simulink library "Lib_Analytic"  (R2019b)
settings: Solver=VariableStepAuto  StartTime=0.0  StopTime=10.0  RelTol=1e-3
undefined symbols (not defined in the file): SJac_Per_M, SNR_DX_M, SNR_IC_M, SNR_Mn_M, SNR_Mx_M
libraries: simulink x2
(part 2 of 2)

== system Lib_Analytic/Solvers/SS NR Solver w JacobianCalc/JacCalc w Reset ==
  f(x) : Inport  PortDimensions=length(SNR_IC_M)
  CCnd : Inport  Port=2  PortDimensions=1
  x(n+1) : Inport  Port=3  PortDimensions=length(SNR_IC_M)
  Enable : EnablePort
  Abs : Abs
  Constant : Constant  Value=SNR_IC_M
  JC_Reset counter : Subsystem
  Jacobian Calculator : Subsystem  TreatAsAtomicUnit=on  mask(T-MATS: Jacobian Calculator Library Block){N_Per_M=SJac_Per_M}
      mask prompts: N_Per_M "N_Per_M - Perturbations (nxm)"
      mask help:
      | The Jacobian Calculator block calculates the Jabobian of the system by perturbing the system around an initial point and calculating the gradient for each perturbation. This module will run once on start up and then again only if the reset is pressed.
      | Below: n (rows) is the number of times each independent will be perturbed and m (columns) is the number of inputs.
      mask Help: web(which('NumMthd_TMATS_JC.html'),'-helpbrowser')
  Product : Product  RndMeth=Zero
  Switch : Switch  Criteria=u2 ~= 0  Threshold=1
  Terminator3 : Terminator
  Unit Delay2 : UnitDelay  InitialCondition=SNR_IC_M./abs(SNR_IC_M)  SampleTime=-1  HasFrameUpgradeWarning=on
  X_out : Outport  PortDimensions=length(SNR_IC_M)
  JC_Active : Outport  Port=2  PortDimensions=1
  inv(J) : Outport  Port=3  PortDimensions=[length(SNR_IC_M),length(SNR_IC_M)]
  J : Outport  Port=4  PortDimensions=[length(SNR_IC_M),length(SNR_IC_M)]
  JacFailed : Outport  Port=5  PortDimensions=1
  wires:
  Jacobian Calculator/3(Iteration) -> Terminator3/1
  Jacobian Calculator/2(x_p) -> Switch/1
  Jacobian Calculator/4(Active) -> [JC_Active], JC_Active/1
  Unit Delay2/1 -> Switch/3, Jacobian Calculator/3(Xo)
  Constant/1 -> Abs/1
  Jacobian Calculator/5(inv(J)) -> inv(J)/1
  [JC_Active] -> JC_Reset counter/1(Reset Counter)
  Switch/1 -> Product/1
  Jacobian Calculator/1(J) -> J/1  "J"
  Product/1 -> X_out/1
  JC_Reset counter/1(JC_Reset) -> Jacobian Calculator/1(Reset)
  x(n+1)/1 -> Unit Delay2/1
  CCnd/1 -> JC_Reset counter/2(Count Condition)
  [JC_Active] -> Switch/2
  f(x)/1 -> Jacobian Calculator/2(f(x_p))
  Jacobian Calculator/6(JacFailed) -> JacFailed/1
  Abs/1 -> Product/2

== system Lib_Analytic/Solvers/SS NR Solver w JacobianCalc/NewRaph w Cond ==
  f(x(n)) : Inport  PortDimensions=length(SNR_IC_M)
  JC_Active : Inport  Port=2  PortDimensions=1
  inv(f'x(n)) : Inport  Port=3  PortDimensions=[length(SNR_IC_M),length(SNR_IC_M)]
  Enable : EnablePort
  Logical Operator : Logic  Operator=NOT  AllPortsSameDT=off  OutDataTypeStr=boolean
  Logical Operator1 : Logic  AllPortsSameDT=off  OutDataTypeStr=boolean
  Logical Operator2 : Logic  Operator=NOT  AllPortsSameDT=off  OutDataTypeStr=boolean
  Newton Raphson Solver : Subsystem  TreatAsAtomicUnit=on  mask(T-MATS: Newton Raphson Solver Library Block){NR_IC_M=SNR_IC_M./abs(SNR_IC_M), NR_dx_Lim_M=SNR_DX_M, NR_Mx_Lim_M=SNR_Mx_M./abs(SNR_IC_M), NR_Mn_Lim_M=SNR_Mn_M./abs(SNR_IC_M), BlkNm_M=double(gcb)}
      mask prompts: NR_IC_M "NR_IC_M - Initial Conditions of Newton Raphson (mx1)"; NR_dx_Lim_M "NR_dx_Lim_M - Newton Raphson step size limit (%) (1x1)"; NR_Mx_Lim_M "NR_Mx_Lim_M - Max limit (1x1 or mx1)"; NR_Mn_Lim_M "NR_Mn_Lim_M - Min Limit (1x1 or mx1)"; BlkNm_M "BlkNm_M - Block Name"
      mask help:
      | Newton Raphson Solver:
      |
      | x(n+1) = x(n) - inverse(f'(x(n)))*f(x(n))
      |
      | Note:
      | inverse(f'(x(n))) is an m x m matrix and f(x(n)) is an m x 1 matrix
      | where m is the length of the initial conditions matrix and number of system independents.
      mask init: same as Lib_Analytic/Numerical Methods/Newton Raphson Solver
      mask Help: web(which('NumMthd_TMATS_NRS.html'),'-helpbrowser')
  Terminator : Terminator
  conditions : Subsystem
  Converged : Outport  PortDimensions={1,[length(SNR_IC_M),length(SNR_IC_M)]}
  CCnd : Outport  Port=2  PortDimensions=1
  x(n+1) : Outport  Port=3  PortDimensions=length(SNR_IC_M)
  wires:
  Logical Operator/1 -> Logical Operator1/1
  Logical Operator1/1 -> Newton Raphson Solver/1(Enable)
  conditions/1(Condition) -> Logical Operator2/1, CCnd/1, Logical Operator1/2
  Logical Operator2/1 -> Converged/1  "Converged"
  JC_Active/1 -> Logical Operator/1
  inv(f'x(n))/1 -> Newton Raphson Solver/2(inv(f'(x(n))))
  Newton Raphson Solver/1(x(n)) -> Terminator/1
  Newton Raphson Solver/2(x(n+1)) -> x(n+1)/1
  f(x(n))/1 -> conditions/1(f(x)), Newton Raphson Solver/3(f(x(n)))

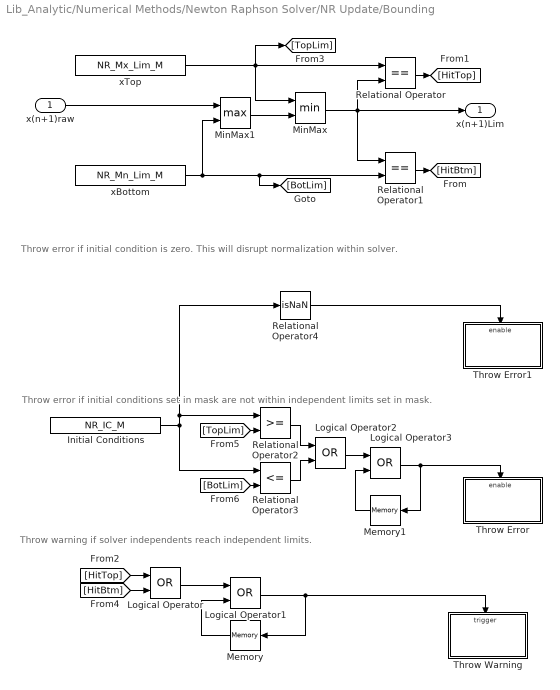
== system Lib_Analytic/Numerical Methods/Newton Raphson Solver/NR Update/Bounding ==
  note: Throw warning if solver independents reach independent limits.
  note: Throw error if initial conditions set in mask are not within independent limits set in mask.
  note: Throw error if initial condition is zero. This will disrupt normalization within solver.
  x(n+1)raw : Inport
  Initial Conditions : Constant  Value=NR_IC_M
  Logical Operator{,1..3} (4 alike) : Logic  Operator=OR  AllPortsSameDT=off  OutDataTypeStr=boolean
  Memory : Memory  InheritSampleTime=on
  Memory1 : Memory  InheritSampleTime=on
  MinMax : MinMax  Inputs=2
  MinMax1 : MinMax  Function=max  Inputs=2
  Relational Operator : RelationalOperator  Operator===  OutDataTypeStr=boolean  RndMeth=Nearest
  Relational Operator1 : RelationalOperator  Operator===  OutDataTypeStr=boolean  RndMeth=Nearest
  Relational Operator2 : RelationalOperator  OutDataTypeStr=boolean  RndMeth=Nearest
  Relational Operator3 : RelationalOperator  Operator=<=  OutDataTypeStr=boolean  RndMeth=Nearest
  Relational Operator4 : RelationalOperator  Operator=isNaN  OutDataTypeStr=boolean  RndMeth=Nearest
  Throw Error : Subsystem
  Throw Error1 : Subsystem
  Throw Warning : Subsystem
  xBottom : Constant  Value=NR_Mn_Lim_M
  xTop : Constant  Value=NR_Mx_Lim_M
  x(n+1)Lim : Outport
  wires:
  Logical Operator1/1 -> Memory/1, Throw Warning/Trigger
  Memory/1 -> Logical Operator1/2
  [HitBtm] -> Logical Operator/2
  Logical Operator/1 -> Logical Operator1/1
  [HitTop] -> Logical Operator/1
  Relational Operator/1 -> [HitTop]
  Relational Operator1/1 -> [HitBtm]
  MinMax/1 -> x(n+1)Lim/1, Relational Operator/2, Relational Operator1/1
  MinMax1/1 -> MinMax/2
  xTop/1 -> [TopLim], MinMax/1, Relational Operator/1
  x(n+1)raw/1 -> MinMax1/1
  xBottom/1 -> [BotLim], Relational Operator1/2, MinMax1/2
  Logical Operator3/1 -> Throw Error/Enable, Memory1/1
  Initial Conditions/1 -> Relational Operator4/1, Relational Operator2/1, Relational Operator3/1
  [TopLim] -> Relational Operator2/2
  Logical Operator2/1 -> Logical Operator3/1
  Relational Operator3/1 -> Logical Operator2/2
  Memory1/1 -> Logical Operator3/2
  Relational Operator2/1 -> Logical Operator2/1
  [BotLim] -> Relational Operator3/2
  Relational Operator4/1 -> Throw Error1/Enable

== system Lib_Analytic/Numerical Methods/Newton Raphson Solver/NR Update/MatrixMult ==
  f(x(n)) : Inport
  inv(f'(x(n))) : Inport  Port=2
  Product : Product  Multiplication=Matrix(*)  RndMeth=Zero
  DTS : Outport
  wires:
  inv(f'(x(n)))/1 -> Product/1
  f(x(n))/1 -> Product/2
  Product/1 -> DTS/1

== system Lib_Analytic/Numerical Methods/Newton Raphson Solver/NR Update/dxLimit ==
  dx : Inport
  x : Inport  Port=2
  Abs : Abs
  Constant : Constant  Value=0.5
  Constant1 : Constant  Value=-1
  Memory : Memory  InitialCondition=NR_IC_M  InheritSampleTime=on
  MinMax : MinMax  Inputs=2
  MinMax1 : MinMax  Function=max  Inputs=2
  Product1 : Product  Inputs=3  RndMeth=Zero
  Product2 : Product  RndMeth=Zero
  Sum : Sum  Inputs=|++
  Threshold : Constant  Value=NR_dx_Lim_M/100
  dx_limited : Outport
  wires:
  Sum/1 -> Product1/3
  Memory/1 -> Sum/1
  Constant/1 -> Product1/2
  x/1 -> Sum/2, Memory/1
  Threshold/1 -> Product1/1
  Product1/1 -> Abs/1
  Abs/1 -> MinMax/1, Product2/2
  dx/1 -> MinMax/2
  MinMax/1 -> MinMax1/2
  Product2/1 -> MinMax1/1
  Constant1/1 -> Product2/1
  MinMax1/1 -> dx_limited/1

== system Lib_Analytic/Solvers/Iterative NR Solver w JacobianCalc/JC w Reset/Jacobian Calculator ==
  Reset : Inport  PortDimensions=1
  f(x_p) : Inport  Port=2  PortDimensions=size(N_Per_M,2)
  Xo : Inport  Port=3  PortDimensions=size(N_Per_M,2)
  Constant2 : Constant  Value=N_Per_M
  Counter : Subsystem  mask{N_Ind_M=prod(size(N_Per_M))}
      mask prompts: N_Ind_M "number of independents, N_Ind_M"
  Jacobian : Subsystem
  Terminator : Terminator
  J : Outport  PortDimensions=[size(N_Per_M,2), size(N_Per_M,2)]
  x_p : Outport  Port=2  PortDimensions=size(N_Per_M,2)
  Iteration : Outport  Port=3  PortDimensions=1
  Active : Outport  Port=4  PortDimensions=1
  inv(J) : Outport  Port=5  PortDimensions=[size(N_Per_M,2), size(N_Per_M,2)]
  JacFailed : Outport  Port=6  PortDimensions=1
  wires:
  Jacobian/5(JacFailed) -> JacFailed/1
  Jacobian/4(y_State) -> Terminator/1
  Jacobian/3(J) -> J/1
  Jacobian/2(Inv(J)) -> inv(J)/1
  Counter/2(Iteration) -> Jacobian/1(Iteration), Iteration/1
  Xo/1 -> Jacobian/4(Xo)
  Counter/1(Enable) -> Jacobian/Enable, Active/1
  Reset/1 -> Counter/1(Reset)
  Jacobian/1(x_p) -> x_p/1
  Constant2/1 -> Jacobian/2(Per)
  f(x_p)/1 -> Jacobian/3(f(x_p))

== system Lib_Analytic/Solvers/Iterative NR Solver w JacobianCalc/NRwCond/Iteration Conditions ==
  f(x) : Inport
  Abs : Abs
  Constant1 : Constant  Value=Cond_Limits_M
  Constant2 : Constant  Value=0
  Relational Operator : RelationalOperator  Operator=>  OutDataTypeStr=boolean  RndMeth=Nearest
  Relational Operator1 : RelationalOperator  Operator=>  OutDataTypeStr=boolean  RndMeth=Nearest
  Sum of Elements : Sum  Inputs=+
  Condition : Outport
  wires:
  Relational Operator1/1 -> Condition/1
  Sum of Elements/1 -> Relational Operator1/1
  Constant2/1 -> Relational Operator1/2
  Relational Operator/1 -> Sum of Elements/1
  f(x)/1 -> Abs/1
  Constant1/1 -> Relational Operator/2
  Abs/1 -> Relational Operator/1

== system Lib_Analytic/Solvers/Iterative NR Solver w JacobianCalc/NRwCond/Newton Raphson Solver ==
  Enable : Inport  PortDimensions=1
  inv(f'(x(n))) : Inport  Port=2  PortDimensions=[length(NR_IC_M),length(NR_IC_M)]
  f(x(n)) : Inport  Port=3  PortDimensions=length(NR_IC_M)
  NR Update : Subsystem
  Switch : Switch  Criteria=u2 > Threshold
  Unit Delay : UnitDelay  InitialCondition=NR_IC_M  SampleTime=-1  HasFrameUpgradeWarning=on
  x(n) : Outport  PortDimensions=length(NR_IC_M)
  x(n+1) : Outport  Port=2  PortDimensions=length(NR_IC_M)
  wires:
  NR Update/1(x(n+1)) -> Switch/1
  inv(f'(x(n)))/1 -> NR Update/2(inv(J))
  f(x(n))/1 -> NR Update/1(f(x))
  Switch/1 -> x(n+1)/1, Unit Delay/1
  Enable/1 -> NR Update/Enable, Switch/2
  Unit Delay/1 -> NR Update/3(x(n)), Switch/3, x(n)/1

== system Lib_Analytic/Solvers/SS NR Solver w JacobianCalc/JacCalc w Reset/JC_Reset counter ==
  Reset Counter : Inport
  Count Condition : Inport  Port=2
  Constant1 : Constant  Value=SJacobianAttempts_M
  Data Type Conversion : DataTypeConversion
  Data Type Conversion1 : DataTypeConversion
  Logical Operator : Logic  Operator=NOT  AllPortsSameDT=off  OutDataTypeStr=boolean
  Product : Product  RndMeth=Zero
  Relational Operator : RelationalOperator  Operator===  OutDataTypeStr=boolean  RndMeth=Nearest
  Sum : Sum  Inputs=|++
  Unit Delay : UnitDelay  SampleTime=-1  HasFrameUpgradeWarning=on
  Unit Delay1 : UnitDelay  SampleTime=-1  HasFrameUpgradeWarning=on
  Unit Delay2 : UnitDelay  SampleTime=-1  HasFrameUpgradeWarning=on
  JC_Reset : Outport
  wires:
  Constant1/1 -> Relational Operator/1
  Relational Operator/1 -> JC_Reset/1
  Product/1 -> Sum/2
  Reset Counter/1 -> Unit Delay1/1
  Unit Delay/1 -> Product/2
  Data Type Conversion/1 -> Product/1
  Data Type Conversion1/1 -> Sum/1
  Unit Delay1/1 -> Logical Operator/1
  Logical Operator/1 -> Data Type Conversion/1
  Count Condition/1 -> Unit Delay2/1
  Unit Delay2/1 -> Data Type Conversion1/1
  Sum/1 -> Unit Delay/1, Relational Operator/2

== system Lib_Analytic/Solvers/SS NR Solver w JacobianCalc/JacCalc w Reset/Jacobian Calculator ==
  Reset : Inport  PortDimensions=1
  f(x_p) : Inport  Port=2  PortDimensions=size(N_Per_M,2)
  Xo : Inport  Port=3  PortDimensions=size(N_Per_M,2)
  Constant2 : Constant  Value=N_Per_M
  Counter : Subsystem  mask{N_Ind_M=prod(size(N_Per_M))}
      mask prompts: N_Ind_M "number of independents, N_Ind_M"
  Jacobian : Subsystem
  Terminator : Terminator
  J : Outport  PortDimensions=[size(N_Per_M,2), size(N_Per_M,2)]
  x_p : Outport  Port=2  PortDimensions=size(N_Per_M,2)
  Iteration : Outport  Port=3  PortDimensions=1
  Active : Outport  Port=4  PortDimensions=1
  inv(J) : Outport  Port=5  PortDimensions=[size(N_Per_M,2), size(N_Per_M,2)]
  JacFailed : Outport  Port=6  PortDimensions=1
  wires:
  Jacobian/5(JacFailed) -> JacFailed/1
  Jacobian/4(y_State) -> Terminator/1
  Jacobian/3(J) -> J/1
  Jacobian/2(Inv(J)) -> inv(J)/1
  Counter/2(Iteration) -> Jacobian/1(Iteration), Iteration/1
  Xo/1 -> Jacobian/4(Xo)
  Counter/1(Enable) -> Jacobian/Enable, Active/1
  Reset/1 -> Counter/1(Reset)
  Jacobian/1(x_p) -> x_p/1
  Constant2/1 -> Jacobian/2(Per)
  f(x_p)/1 -> Jacobian/3(f(x_p))

== system Lib_Analytic/Solvers/SS NR Solver w JacobianCalc/NewRaph w Cond/Newton Raphson Solver ==
  Enable : Inport  PortDimensions=1
  inv(f'(x(n))) : Inport  Port=2  PortDimensions=[length(NR_IC_M),length(NR_IC_M)]
  f(x(n)) : Inport  Port=3  PortDimensions=length(NR_IC_M)
  NR Update : Subsystem
  Switch : Switch  Criteria=u2 > Threshold
  Unit Delay : UnitDelay  InitialCondition=NR_IC_M  SampleTime=-1  HasFrameUpgradeWarning=on
  x(n) : Outport  PortDimensions=length(NR_IC_M)
  x(n+1) : Outport  Port=2  PortDimensions=length(NR_IC_M)
  wires:
  NR Update/1(x(n+1)) -> Switch/1
  inv(f'(x(n)))/1 -> NR Update/2(inv(J))
  f(x(n))/1 -> NR Update/1(f(x))
  Switch/1 -> x(n+1)/1, Unit Delay/1
  Enable/1 -> NR Update/Enable, Switch/2
  Unit Delay/1 -> NR Update/3(x(n)), Switch/3, x(n)/1

== system Lib_Analytic/Solvers/SS NR Solver w JacobianCalc/NewRaph w Cond/conditions ==
  f(x) : Inport
  Abs : Abs
  Constant2 : Constant  Value=Cond_Limits_M
  Constant3 : Constant  Value=0
  Relational Operator1 : RelationalOperator  Operator=>  OutDataTypeStr=boolean  RndMeth=Nearest
  Relational Operator2 : RelationalOperator  Operator=>  OutDataTypeStr=boolean  RndMeth=Nearest
  Sum of Elements : Sum  Inputs=+
  Condition : Outport
  wires:
  Constant2/1 -> Relational Operator1/2
  Relational Operator1/1 -> Sum of Elements/1
  Constant3/1 -> Relational Operator2/2
  Abs/1 -> Relational Operator1/1
  Sum of Elements/1 -> Relational Operator2/1
  f(x)/1 -> Abs/1
  Relational Operator2/1 -> Condition/1

== system Lib_Analytic/Numerical Methods/Newton Raphson Solver/NR Update/Bounding/Throw Error ==
  Enable : EnablePort
  MATLAB Function : MATLAB Function  TreatAsAtomicUnit=on

== system Lib_Analytic/Numerical Methods/Newton Raphson Solver/NR Update/Bounding/Throw Error1 ==
  Enable : EnablePort
  MATLAB Function : MATLAB Function  TreatAsAtomicUnit=on

== system Lib_Analytic/Numerical Methods/Newton Raphson Solver/NR Update/Bounding/Throw Warning ==
  Trigger : TriggerPort  VariantControl=(inherit)
  MATLAB Function : MATLAB Function  TreatAsAtomicUnit=on

== system Lib_Analytic/Solvers/Iterative NR Solver w JacobianCalc/JC w Reset/Jacobian Calculator/Counter ==
  Reset : Inport
  Constant : Constant
  Constant1 : Constant  Value=N_Ind_M
  Constant2 : Constant  Value=3
  Logical Operator1 : Logic  Operator=NOT  AllPortsSameDT=off  OutDataTypeStr=boolean
  MinMax1 : MinMax  Inputs=2
  Product : Product  RndMeth=Zero
  Relational Operator : RelationalOperator  Operator=>  OutDataTypeStr=boolean  RndMeth=Nearest
  Sum : Sum  Inputs=|++
  Sum1 : Sum  Inputs=|++
  Unit Delay : UnitDelay  SampleTime=-1  HasFrameUpgradeWarning=on
  Enable : Outport
  Iteration : Outport  Port=2
  wires:
  Constant1/1 -> Sum1/1
  Constant2/1 -> Sum1/2
  Sum1/1 -> Product/1, Relational Operator/1
  Reset/1 -> Logical Operator1/1
  Logical Operator1/1 -> Product/2
  Relational Operator/1 -> Enable/1
  MinMax1/1 -> Relational Operator/2, Iteration/1, Unit Delay/1
  Unit Delay/1 -> Sum/2
  Sum/1 -> MinMax1/2
  Product/1 -> MinMax1/1
  Constant/1 -> Sum/1

== system Lib_Analytic/Solvers/Iterative NR Solver w JacobianCalc/JC w Reset/Jacobian Calculator/Jacobian ==
  Iteration : Inport
  Per : Inport  Port=2
  f(x_p) : Inport  Port=3
  Xo : Inport  Port=4
  Enable : EnablePort
  Jacobian Calc : MATLAB Function  TreatAsAtomicUnit=on
  Unit Delay : UnitDelay  InitialCondition=zeros(size(N_Per_M,2),size(N_Per_M,2))  SampleTime=-1  HasFrameUpgradeWarning=on
  Unit Delay1 : UnitDelay  InitialCondition=zeros(size(N_Per_M,2),prod(size(N_Per_M))+1)  SampleTime=-1  HasFrameUpgradeWarning=on
  Unit Delay2 : UnitDelay  InitialCondition=zeros(size(N_Per_M,2),1)  SampleTime=-1  HasFrameUpgradeWarning=on
  Unit Delay3 : UnitDelay  SampleTime=-1  HasFrameUpgradeWarning=on
  x_p : Outport
  Inv(J) : Outport  Port=2
  J : Outport  Port=3
  y_State : Outport  Port=4
  JacFailed : Outport  Port=5
  wires:
  Unit Delay3/1 -> Jacobian Calc/7(Er)
  Jacobian Calc/5(ErSv) -> JacFailed/1, Unit Delay3/1
  Unit Delay2/1 -> Jacobian Calc/2(y_xpIn)
  f(x_p)/1 -> Unit Delay2/1
  Unit Delay1/1 -> Jacobian Calc/6(y_StateIn)
  Jacobian Calc/4(y_StateOut) -> y_State/1, Unit Delay1/1
  Unit Delay/1 -> Jacobian Calc/5(JStateIn)
  Jacobian Calc/2(InvJOut) -> Inv(J)/1
  Jacobian Calc/3(JOut) -> J/1, Unit Delay/1
  Iteration/1 -> Jacobian Calc/1(IterationIn)
  Per/1 -> Jacobian Calc/3(PerIn)
  Xo/1 -> Jacobian Calc/4(XoIn)
  Jacobian Calc/1(XpOut) -> x_p/1

== system Lib_Analytic/Solvers/Iterative NR Solver w JacobianCalc/NRwCond/Newton Raphson Solver/NR Update ==
  f(x) : Inport
  inv(J) : Inport  Port=2
  x(n) : Inport  Port=3
  Enable : EnablePort
  Bounding : Subsystem
  MatrixMult : Subsystem
  Sum : Sum  Inputs=|-+
  dxLimit : Subsystem
  x(n+1) : Outport
  wires:
  x(n)/1 -> Sum/2, dxLimit/2(x)
  Bounding/1(x(n+1)Lim) -> x(n+1)/1
  inv(J)/1 -> MatrixMult/2(inv(f'(x(n))))
  dxLimit/1(dx_limited) -> Sum/1
  MatrixMult/1(DTS) -> dxLimit/1(dx)
  Sum/1 -> Bounding/1(x(n+1)raw)
  f(x)/1 -> MatrixMult/1(f(x(n)))

== system Lib_Analytic/Solvers/SS NR Solver w JacobianCalc/JacCalc w Reset/Jacobian Calculator/Counter ==
  Reset : Inport
  Constant : Constant
  Constant1 : Constant  Value=N_Ind_M
  Constant2 : Constant  Value=3
  Logical Operator1 : Logic  Operator=NOT  AllPortsSameDT=off  OutDataTypeStr=boolean
  MinMax1 : MinMax  Inputs=2
  Product : Product  RndMeth=Zero
  Relational Operator : RelationalOperator  Operator=>  OutDataTypeStr=boolean  RndMeth=Nearest
  Sum : Sum  Inputs=|++
  Sum1 : Sum  Inputs=|++
  Unit Delay : UnitDelay  SampleTime=-1  HasFrameUpgradeWarning=on
  Enable : Outport
  Iteration : Outport  Port=2
  wires:
  Constant1/1 -> Sum1/1
  Constant2/1 -> Sum1/2
  Sum1/1 -> Product/1, Relational Operator/1
  Reset/1 -> Logical Operator1/1
  Logical Operator1/1 -> Product/2
  Relational Operator/1 -> Enable/1
  MinMax1/1 -> Relational Operator/2, Iteration/1, Unit Delay/1
  Unit Delay/1 -> Sum/2
  Sum/1 -> MinMax1/2
  Product/1 -> MinMax1/1
  Constant/1 -> Sum/1

== system Lib_Analytic/Solvers/SS NR Solver w JacobianCalc/JacCalc w Reset/Jacobian Calculator/Jacobian ==
  Iteration : Inport
  Per : Inport  Port=2
  f(x_p) : Inport  Port=3
  Xo : Inport  Port=4
  Enable : EnablePort
  Jacobian Calc : MATLAB Function  TreatAsAtomicUnit=on
  Unit Delay : UnitDelay  InitialCondition=zeros(size(N_Per_M,2),size(N_Per_M,2))  SampleTime=-1  HasFrameUpgradeWarning=on
  Unit Delay1 : UnitDelay  InitialCondition=zeros(size(N_Per_M,2),prod(size(N_Per_M))+1)  SampleTime=-1  HasFrameUpgradeWarning=on
  Unit Delay2 : UnitDelay  InitialCondition=zeros(size(N_Per_M,2),1)  SampleTime=-1  HasFrameUpgradeWarning=on
  Unit Delay3 : UnitDelay  SampleTime=-1  HasFrameUpgradeWarning=on
  x_p : Outport
  Inv(J) : Outport  Port=2
  J : Outport  Port=3
  y_State : Outport  Port=4
  JacFailed : Outport  Port=5
  wires:
  Unit Delay3/1 -> Jacobian Calc/7(Er)
  Jacobian Calc/5(ErSv) -> JacFailed/1, Unit Delay3/1
  Unit Delay2/1 -> Jacobian Calc/2(y_xpIn)
  f(x_p)/1 -> Unit Delay2/1
  Unit Delay1/1 -> Jacobian Calc/6(y_StateIn)
  Jacobian Calc/4(y_StateOut) -> y_State/1, Unit Delay1/1
  Unit Delay/1 -> Jacobian Calc/5(JStateIn)
  Jacobian Calc/2(InvJOut) -> Inv(J)/1
  Jacobian Calc/3(JOut) -> J/1, Unit Delay/1
  Iteration/1 -> Jacobian Calc/1(IterationIn)
  Per/1 -> Jacobian Calc/3(PerIn)
  Xo/1 -> Jacobian Calc/4(XoIn)
  Jacobian Calc/1(XpOut) -> x_p/1

== system Lib_Analytic/Solvers/SS NR Solver w JacobianCalc/NewRaph w Cond/Newton Raphson Solver/NR Update ==
  f(x) : Inport
  inv(J) : Inport  Port=2
  x(n) : Inport  Port=3
  Enable : EnablePort
  Bounding : Subsystem
  MatrixMult : Subsystem
  Sum : Sum  Inputs=|-+
  dxLimit : Subsystem
  x(n+1) : Outport
  wires:
  x(n)/1 -> Sum/2, dxLimit/2(x)
  Bounding/1(x(n+1)Lim) -> x(n+1)/1
  inv(J)/1 -> MatrixMult/2(inv(f'(x(n))))
  dxLimit/1(dx_limited) -> Sum/1
  MatrixMult/1(DTS) -> dxLimit/1(dx)
  Sum/1 -> Bounding/1(x(n+1)raw)
  f(x)/1 -> MatrixMult/1(f(x(n)))

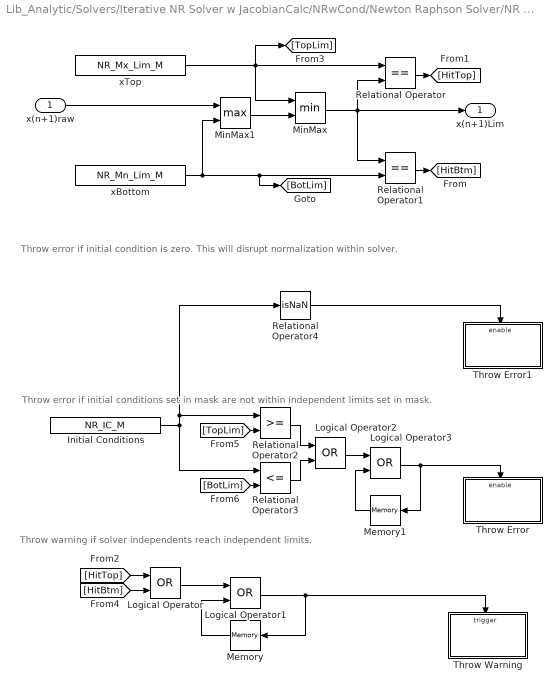
== system Lib_Analytic/Solvers/Iterative NR Solver w JacobianCalc/NRwCond/Newton Raphson Solver/NR Update/Bounding ==
  note: Throw warning if solver independents reach independent limits.
  note: Throw error if initial conditions set in mask are not within independent limits set in mask.
  note: Throw error if initial condition is zero. This will disrupt normalization within solver.
  x(n+1)raw : Inport
  Initial Conditions : Constant  Value=NR_IC_M
  Logical Operator{,1..3} (4 alike) : Logic  Operator=OR  AllPortsSameDT=off  OutDataTypeStr=boolean
  Memory : Memory  InheritSampleTime=on
  Memory1 : Memory  InheritSampleTime=on
  MinMax : MinMax  Inputs=2
  MinMax1 : MinMax  Function=max  Inputs=2
  Relational Operator : RelationalOperator  Operator===  OutDataTypeStr=boolean  RndMeth=Nearest
  Relational Operator1 : RelationalOperator  Operator===  OutDataTypeStr=boolean  RndMeth=Nearest
  Relational Operator2 : RelationalOperator  OutDataTypeStr=boolean  RndMeth=Nearest
  Relational Operator3 : RelationalOperator  Operator=<=  OutDataTypeStr=boolean  RndMeth=Nearest
  Relational Operator4 : RelationalOperator  Operator=isNaN  OutDataTypeStr=boolean  RndMeth=Nearest
  Throw Error : Subsystem
  Throw Error1 : Subsystem
  Throw Warning : Subsystem
  xBottom : Constant  Value=NR_Mn_Lim_M
  xTop : Constant  Value=NR_Mx_Lim_M
  x(n+1)Lim : Outport
  wires:
  Logical Operator1/1 -> Memory/1, Throw Warning/Trigger
  Memory/1 -> Logical Operator1/2
  [HitBtm] -> Logical Operator/2
  Logical Operator/1 -> Logical Operator1/1
  [HitTop] -> Logical Operator/1
  Relational Operator/1 -> [HitTop]
  Relational Operator1/1 -> [HitBtm]
  MinMax/1 -> x(n+1)Lim/1, Relational Operator/2, Relational Operator1/1
  MinMax1/1 -> MinMax/2
  xTop/1 -> [TopLim], MinMax/1, Relational Operator/1
  x(n+1)raw/1 -> MinMax1/1
  xBottom/1 -> [BotLim], Relational Operator1/2, MinMax1/2
  Logical Operator3/1 -> Throw Error/Enable, Memory1/1
  Initial Conditions/1 -> Relational Operator4/1, Relational Operator2/1, Relational Operator3/1
  [TopLim] -> Relational Operator2/2
  Logical Operator2/1 -> Logical Operator3/1
  Relational Operator3/1 -> Logical Operator2/2
  Memory1/1 -> Logical Operator3/2
  Relational Operator2/1 -> Logical Operator2/1
  [BotLim] -> Relational Operator3/2
  Relational Operator4/1 -> Throw Error1/Enable

== system Lib_Analytic/Solvers/Iterative NR Solver w JacobianCalc/NRwCond/Newton Raphson Solver/NR Update/MatrixMult ==
  f(x(n)) : Inport
  inv(f'(x(n))) : Inport  Port=2
  Product : Product  Multiplication=Matrix(*)  RndMeth=Zero
  DTS : Outport
  wires:
  inv(f'(x(n)))/1 -> Product/1
  f(x(n))/1 -> Product/2
  Product/1 -> DTS/1

== system Lib_Analytic/Solvers/Iterative NR Solver w JacobianCalc/NRwCond/Newton Raphson Solver/NR Update/dxLimit ==
  dx : Inport
  x : Inport  Port=2
  Abs : Abs
  Constant : Constant  Value=0.5
  Constant1 : Constant  Value=-1
  Memory : Memory  InitialCondition=NR_IC_M  InheritSampleTime=on
  MinMax : MinMax  Inputs=2
  MinMax1 : MinMax  Function=max  Inputs=2
  Product1 : Product  Inputs=3  RndMeth=Zero
  Product2 : Product  RndMeth=Zero
  Sum : Sum  Inputs=|++
  Threshold : Constant  Value=NR_dx_Lim_M/100
  dx_limited : Outport
  wires:
  Sum/1 -> Product1/3
  Memory/1 -> Sum/1
  Constant/1 -> Product1/2
  x/1 -> Sum/2, Memory/1
  Threshold/1 -> Product1/1
  Product1/1 -> Abs/1
  Abs/1 -> MinMax/1, Product2/2
  dx/1 -> MinMax/2
  MinMax/1 -> MinMax1/2
  Product2/1 -> MinMax1/1
  Constant1/1 -> Product2/1
  MinMax1/1 -> dx_limited/1

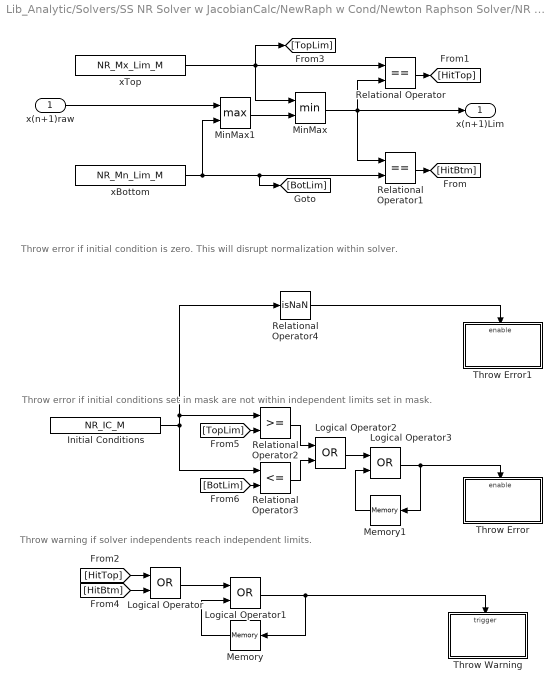
== system Lib_Analytic/Solvers/SS NR Solver w JacobianCalc/NewRaph w Cond/Newton Raphson Solver/NR Update/Bounding ==
  note: Throw warning if solver independents reach independent limits.
  note: Throw error if initial conditions set in mask are not within independent limits set in mask.
  note: Throw error if initial condition is zero. This will disrupt normalization within solver.
  x(n+1)raw : Inport
  Initial Conditions : Constant  Value=NR_IC_M
  Logical Operator{,1..3} (4 alike) : Logic  Operator=OR  AllPortsSameDT=off  OutDataTypeStr=boolean
  Memory : Memory  InheritSampleTime=on
  Memory1 : Memory  InheritSampleTime=on
  MinMax : MinMax  Inputs=2
  MinMax1 : MinMax  Function=max  Inputs=2
  Relational Operator : RelationalOperator  Operator===  OutDataTypeStr=boolean  RndMeth=Nearest
  Relational Operator1 : RelationalOperator  Operator===  OutDataTypeStr=boolean  RndMeth=Nearest
  Relational Operator2 : RelationalOperator  OutDataTypeStr=boolean  RndMeth=Nearest
  Relational Operator3 : RelationalOperator  Operator=<=  OutDataTypeStr=boolean  RndMeth=Nearest
  Relational Operator4 : RelationalOperator  Operator=isNaN  OutDataTypeStr=boolean  RndMeth=Nearest
  Throw Error : Subsystem
  Throw Error1 : Subsystem
  Throw Warning : Subsystem
  xBottom : Constant  Value=NR_Mn_Lim_M
  xTop : Constant  Value=NR_Mx_Lim_M
  x(n+1)Lim : Outport
  wires:
  Logical Operator1/1 -> Memory/1, Throw Warning/Trigger
  Memory/1 -> Logical Operator1/2
  [HitBtm] -> Logical Operator/2
  Logical Operator/1 -> Logical Operator1/1
  [HitTop] -> Logical Operator/1
  Relational Operator/1 -> [HitTop]
  Relational Operator1/1 -> [HitBtm]
  MinMax/1 -> x(n+1)Lim/1, Relational Operator/2, Relational Operator1/1
  MinMax1/1 -> MinMax/2
  xTop/1 -> [TopLim], MinMax/1, Relational Operator/1
  x(n+1)raw/1 -> MinMax1/1
  xBottom/1 -> [BotLim], Relational Operator1/2, MinMax1/2
  Logical Operator3/1 -> Throw Error/Enable, Memory1/1
  Initial Conditions/1 -> Relational Operator4/1, Relational Operator2/1, Relational Operator3/1
  [TopLim] -> Relational Operator2/2
  Logical Operator2/1 -> Logical Operator3/1
  Relational Operator3/1 -> Logical Operator2/2
  Memory1/1 -> Logical Operator3/2
  Relational Operator2/1 -> Logical Operator2/1
  [BotLim] -> Relational Operator3/2
  Relational Operator4/1 -> Throw Error1/Enable

== system Lib_Analytic/Solvers/SS NR Solver w JacobianCalc/NewRaph w Cond/Newton Raphson Solver/NR Update/MatrixMult ==
  f(x(n)) : Inport
  inv(f'(x(n))) : Inport  Port=2
  Product : Product  Multiplication=Matrix(*)  RndMeth=Zero
  DTS : Outport
  wires:
  inv(f'(x(n)))/1 -> Product/1
  f(x(n))/1 -> Product/2
  Product/1 -> DTS/1

== system Lib_Analytic/Solvers/SS NR Solver w JacobianCalc/NewRaph w Cond/Newton Raphson Solver/NR Update/dxLimit ==
  dx : Inport
  x : Inport  Port=2
  Abs : Abs
  Constant : Constant  Value=0.5
  Constant1 : Constant  Value=-1
  Memory : Memory  InitialCondition=NR_IC_M  InheritSampleTime=on
  MinMax : MinMax  Inputs=2
  MinMax1 : MinMax  Function=max  Inputs=2
  Product1 : Product  Inputs=3  RndMeth=Zero
  Product2 : Product  RndMeth=Zero
  Sum : Sum  Inputs=|++
  Threshold : Constant  Value=NR_dx_Lim_M/100
  dx_limited : Outport
  wires:
  Sum/1 -> Product1/3
  Memory/1 -> Sum/1
  Constant/1 -> Product1/2
  x/1 -> Sum/2, Memory/1
  Threshold/1 -> Product1/1
  Product1/1 -> Abs/1
  Abs/1 -> MinMax/1, Product2/2
  dx/1 -> MinMax/2
  MinMax/1 -> MinMax1/2
  Product2/1 -> MinMax1/1
  Constant1/1 -> Product2/1
  MinMax1/1 -> dx_limited/1

== system Lib_Analytic/Solvers/Iterative NR Solver w JacobianCalc/NRwCond/Newton Raphson Solver/NR Update/Bounding/Throw Error ==
  Enable : EnablePort
  MATLAB Function : MATLAB Function  TreatAsAtomicUnit=on

== system Lib_Analytic/Solvers/Iterative NR Solver w JacobianCalc/NRwCond/Newton Raphson Solver/NR Update/Bounding/Throw Error1 ==
  Enable : EnablePort
  MATLAB Function : MATLAB Function  TreatAsAtomicUnit=on

== system Lib_Analytic/Solvers/Iterative NR Solver w JacobianCalc/NRwCond/Newton Raphson Solver/NR Update/Bounding/Throw Warning ==
  Trigger : TriggerPort  VariantControl=(inherit)
  MATLAB Function : MATLAB Function  TreatAsAtomicUnit=on

== system Lib_Analytic/Solvers/SS NR Solver w JacobianCalc/NewRaph w Cond/Newton Raphson Solver/NR Update/Bounding/Throw Error ==
  Enable : EnablePort
  MATLAB Function : MATLAB Function  TreatAsAtomicUnit=on

== system Lib_Analytic/Solvers/SS NR Solver w JacobianCalc/NewRaph w Cond/Newton Raphson Solver/NR Update/Bounding/Throw Error1 ==
  Enable : EnablePort
  MATLAB Function : MATLAB Function  TreatAsAtomicUnit=on

== system Lib_Analytic/Solvers/SS NR Solver w JacobianCalc/NewRaph w Cond/Newton Raphson Solver/NR Update/Bounding/Throw Warning ==
  Trigger : TriggerPort  VariantControl=(inherit)
  MATLAB Function : MATLAB Function  TreatAsAtomicUnit=on

== matlab function Lib_Analytic/Numerical Methods/Jacobian Calculator/Jacobian/Jacobian Calc ==
  data: IterationIn input; XpOut output; y_xpIn input; PerIn input; XoIn input; InvJOut output; JOut output; JStateIn input; y_StateIn input; y_StateOut output; Er input; ErSv output
function [XpOut, InvJOut, JOut, y_StateOut, ErSv] = fcn(IterationIn, y_xpIn, PerIn, XoIn, JStateIn, y_StateIn, Er)

% Set inital condiations
i = IterationIn;
XpOut = XoIn;
InvJOut = zeros(length(XoIn));
JOut = JStateIn;
y_StateOut = y_StateIn;
PerVec = reshape(PerIn',1,[]);
LenPV = length(PerVec);
LenXo = length(XoIn);
ErSv = Er;

% Begin taking data from f(x) at iteration a+1
a = 1;
% Begin determining Jacobian at iteration b+1
b = a+1;

% Set Xp Output
if i > a && i <= LenPV + a
    current_Xp = mod(i-a-1,LenXo)+1;
    XpOut(current_Xp) = XpOut(current_Xp) + PerVec(i - a);
end

% save state feedback
if LenXo == 1
    if i >= b;
        y_StateOut(i-a) = y_xpIn;
    end
else
    if i > a && i<= LenPV + a+1;
        y_StateOut(:,i - a) = y_xpIn;
    end
end

% Create Jacobian
if i == LenPV + b
    % Generate Jacobian matrices for each set, stacked.
    if LenXo == 1
        JMtx_extended = (y_StateOut(2:end)' - repmat(y_StateOut(1),1,LenPV))./PerVec;
    else
        JMtx_extended = (y_StateOut(:,2:end) - repmat(y_StateOut(:,1),1,LenPV))./repmat(PerVec,LenXo,1);
    end
    
    % Initialize sum matricies
    JMtrx_sum = zeros(LenXo);
    Nsum = zeros(LenXo);
    
    % determine how many perturbation sets there are, b/c MATLAB likes to
    % flip vectors when they enter MATLAB functions from Simulink for no reason.
    if min(size(PerIn)) == 1
     if LenXo == 1;
        PerNum = length(PerIn); 
     else 
        PerNum = 1;
     end
    else
        PerNum = size(PerIn,1);
    end
    
    for set = 1: PerNum
        % Break out Jacobian matrix for the current perturbation set
        JMtrx_cur = JMtx_extended(:, LenXo*(set-1)+1:LenXo*set);
        % Sum Jacobian matrices for each set
        JMtrx_sum = JMtrx_sum + JMtrx_cur(:,1:LenXo);
        % Sum number of acceptable values
        Nsum = Nsum + abs(sign(JMtrx_cur(:,1:LenXo)));
    end
    
    % Average Jacobian Matricies
    Javg = JMtrx_sum./max(Nsum,1);
    
    JOut = Javg;
    
    % Invert Jacobian
    if rank(JOut) == length(InvJOut)
        InvJOut = inv(JOut(:,:));
    elseif ErSv < 1
        disp('Jacobian can not be inverted.');
        ErSv = 1;
    end
end

== matlab function Lib_Analytic/Numerical Methods/Newton Raphson Solver/NR Update/Bounding/Throw Error/MATLAB Function ==
  data: BlkNm_M parameter
function ICNotInsideLimits(BlkNm_M)
%# Throw error if initial condition is outside bounds on independent.
BName = BlkNm_M;
error(['Error in ' BName ': Initial conditions, SNR_IC_M, of NR Solver are not within the Newton Raphson independent limits, SNR_Mx_M and SNR_Mn_M. Please choose initial condiitons conditions within the prescribed limits.']);

== matlab function Lib_Analytic/Numerical Methods/Newton Raphson Solver/NR Update/Bounding/Throw Error1/MATLAB Function ==
  data: BlkNm_M parameter
function ICIsZero(BlkNm_M)
%# Throw error if initial condition is outside bounds on independent.
BName = BlkNm_M;
error(['Error in ' BName ': Initial conditions, SNR_IC_M, of NR Solver are zero. This will disrupt the normalization within the solver. Please choose non-zero numbers.']);

== matlab function Lib_Analytic/Solvers/SS NR Solver w JacobianCalc/JacCalc w Reset/Jacobian Calculator/Jacobian/Jacobian Calc ==
  data: IterationIn input; XpOut output; y_xpIn input; PerIn input; XoIn input; InvJOut output; JOut output; JStateIn input; y_StateIn input; y_StateOut output; Er input; ErSv output
function [XpOut, InvJOut, JOut, y_StateOut, ErSv] = fcn(IterationIn, y_xpIn, PerIn, XoIn, JStateIn, y_StateIn, Er)

% Set inital condiations
i = IterationIn;
XpOut = XoIn;
InvJOut = zeros(length(XoIn));
JOut = JStateIn;
y_StateOut = y_StateIn;
PerVec = reshape(PerIn',1,[]);
LenPV = length(PerVec);
LenXo = length(XoIn);
ErSv = Er;

% Begin taking data from f(x) at iteration a+1
a = 1;
% Begin determining Jacobian at iteration b+1
b = a+1;

% Set Xp Output
if i > a && i <= LenPV + a
    current_Xp = mod(i-a-1,LenXo)+1;
    XpOut(current_Xp) = XpOut(current_Xp) + PerVec(i - a);
end

% save state feedback
if LenXo == 1
    if i >= b;
        y_StateOut(i-a) = y_xpIn;
    end
else
    if i > a && i<= LenPV + a+1;
        y_StateOut(:,i - a) = y_xpIn;
    end
end

% Create Jacobian
if i == LenPV + b
    % Generate Jacobian matrices for each set, stacked.
    if LenXo == 1
        JMtx_extended = (y_StateOut(2:end)' - repmat(y_StateOut(1),1,LenPV))./PerVec;
    else
        JMtx_extended = (y_StateOut(:,2:end) - repmat(y_StateOut(:,1),1,LenPV))./repmat(PerVec,LenXo,1);
    end
    
    % Initialize sum matricies
    JMtrx_sum = zeros(LenXo);
    Nsum = zeros(LenXo);
    
    % determine how many perturbation sets there are, b/c MATLAB likes to
    % flip vectors when they enter MATLAB functions from Simulink for no reason.
    if min(size(PerIn)) == 1
     if LenXo == 1;
        PerNum = length(PerIn); 
     else 
        PerNum = 1;
     end
    else
        PerNum = size(PerIn,1);
    end
    
    for set = 1: PerNum
        % Break out Jacobian matrix for the current perturbation set
        JMtrx_cur = JMtx_extended(:, LenXo*(set-1)+1:LenXo*set);
        % Sum Jacobian matrices for each set
        JMtrx_sum = JMtrx_sum + JMtrx_cur(:,1:LenXo);
        % Sum number of acceptable values
        Nsum = Nsum + abs(sign(JMtrx_cur(:,1:LenXo)));
    end
    
    % Average Jacobian Matricies
    Javg = JMtrx_sum./max(Nsum,1);
    
    JOut = Javg;
    
    % Invert Jacobian
    if rank(JOut) == length(InvJOut)
        InvJOut = inv(JOut(:,:));
    elseif ErSv < 1
        disp('Jacobian can not be inverted.');
        ErSv = 1;
    end
end

== matlab function Lib_Analytic/Solvers/SS NR Solver w JacobianCalc/NewRaph w Cond/Newton Raphson Solver/NR Update/Bounding/Throw Warning/MATLAB Function ==
  data: BlkNm_M parameter
function fcn(BlkNm_M)
%# Limit Newton Raphson outputs and produce a warning if it occurs
BName = BlkNm_M;
disp(['Warning in ' BName ': Solver limit has been hit, check for system convergence']);

== matlab function Lib_Analytic/Numerical Methods/Newton Raphson Solver/NR Update/Bounding/Throw Warning/MATLAB Function ==
  data: BlkNm_M parameter
function fcn(BlkNm_M)
%# Limit Newton Raphson outputs and produce a warning if it occurs
BName = BlkNm_M;
disp(['Warning in ' BName ': Solver limit has been hit, check for system convergence']);

== matlab function Lib_Analytic/Solvers/Iterative NR Solver w JacobianCalc/JC w Reset/Jacobian Calculator/Jacobian/Jacobian Calc ==
  data: IterationIn input; XpOut output; y_xpIn input; PerIn input; XoIn input; InvJOut output; JOut output; JStateIn input; y_StateIn input; y_StateOut output; Er input; ErSv output
function [XpOut, InvJOut, JOut, y_StateOut, ErSv] = fcn(IterationIn, y_xpIn, PerIn, XoIn, JStateIn, y_StateIn, Er)

% Set inital condiations
i = IterationIn;
XpOut = XoIn;
InvJOut = zeros(length(XoIn));
JOut = JStateIn;
y_StateOut = y_StateIn;
PerVec = reshape(PerIn',1,[]);
LenPV = length(PerVec);
LenXo = length(XoIn);
ErSv = Er;

% Begin taking data from f(x) at iteration a+1
a = 1;
% Begin determining Jacobian at iteration b+1
b = a+1;

% Set Xp Output
if i > a && i <= LenPV + a
    current_Xp = mod(i-a-1,LenXo)+1;
    XpOut(current_Xp) = XpOut(current_Xp) + PerVec(i - a);
end

% save state feedback
if LenXo == 1
    if i >= b;
        y_StateOut(i-a) = y_xpIn;
    end
else
    if i > a && i<= LenPV + a+1;
        y_StateOut(:,i - a) = y_xpIn;
    end
end

% Create Jacobian
if i == LenPV + b
    % Generate Jacobian matrices for each set, stacked.
    if LenXo == 1
        JMtx_extended = (y_StateOut(2:end)' - repmat(y_StateOut(1),1,LenPV))./PerVec;
    else
        JMtx_extended = (y_StateOut(:,2:end) - repmat(y_StateOut(:,1),1,LenPV))./repmat(PerVec,LenXo,1);
    end
    
    % Initialize sum matricies
    JMtrx_sum = zeros(LenXo);
    Nsum = zeros(LenXo);
    
    % determine how many perturbation sets there are, b/c MATLAB likes to
    % flip vectors when they enter MATLAB functions from Simulink for no reason.
    if min(size(PerIn)) == 1
     if LenXo == 1;
        PerNum = length(PerIn); 
     else 
        PerNum = 1;
     end
    else
        PerNum = size(PerIn,1);
    end
    
    for set = 1: PerNum
        % Break out Jacobian matrix for the current perturbation set
        JMtrx_cur = JMtx_extended(:, LenXo*(set-1)+1:LenXo*set);
        % Sum Jacobian matrices for each set
        JMtrx_sum = JMtrx_sum + JMtrx_cur(:,1:LenXo);
        % Sum number of acceptable values
        Nsum = Nsum + abs(sign(JMtrx_cur(:,1:LenXo)));
    end
    
    % Average Jacobian Matricies
    Javg = JMtrx_sum./max(Nsum,1);
    
    JOut = Javg;
    
    % Invert Jacobian
    if rank(JOut) == length(InvJOut)
        InvJOut = inv(JOut(:,:));
    elseif ErSv < 1
        disp('Jacobian can not be inverted.');
        ErSv = 1;
    end
end

== matlab function Lib_Analytic/Solvers/Iterative NR Solver w JacobianCalc/NRwCond/Newton Raphson Solver/NR Update/Bounding/Throw Error/MATLAB Function ==
  data: BlkNm_M parameter
function ICNotInsideLimits(BlkNm_M)
%# Throw error if initial condition is outside bounds on independent.
BName = BlkNm_M;
error(['Error in ' BName ': Initial conditions, SNR_IC_M, of NR Solver are not within the Newton Raphson independent limits, SNR_Mx_M and SNR_Mn_M. Please choose initial condiitons conditions within the prescribed limits.']);

== matlab function Lib_Analytic/Solvers/Iterative NR Solver w JacobianCalc/NRwCond/Newton Raphson Solver/NR Update/Bounding/Throw Error1/MATLAB Function ==
  data: BlkNm_M parameter
function ICIsZero(BlkNm_M)
%# Throw error if initial condition is outside bounds on independent.
BName = BlkNm_M;
error(['Error in ' BName ': Initial conditions, SNR_IC_M, of NR Solver are zero. This will disrupt the normalization within the solver. Please choose non-zero numbers.']);

== matlab function Lib_Analytic/Solvers/SS NR Solver w JacobianCalc/NewRaph w Cond/Newton Raphson Solver/NR Update/Bounding/Throw Error/MATLAB Function ==
  data: BlkNm_M parameter
function ICNotInsideLimits(BlkNm_M)
%# Throw error if initial condition is outside bounds on independent.
BName = BlkNm_M;
error(['Error in ' BName ': Initial conditions, SNR_IC_M, of NR Solver are not within the Newton Raphson independent limits, SNR_Mx_M and SNR_Mn_M. Please choose initial condiitons conditions within the prescribed limits.']);

== matlab function Lib_Analytic/Solvers/SS NR Solver w JacobianCalc/NewRaph w Cond/Newton Raphson Solver/NR Update/Bounding/Throw Error1/MATLAB Function ==
  data: BlkNm_M parameter
function ICIsZero(BlkNm_M)
%# Throw error if initial condition is outside bounds on independent.
BName = BlkNm_M;
error(['Error in ' BName ': Initial conditions, SNR_IC_M, of NR Solver are zero. This will disrupt the normalization within the solver. Please choose non-zero numbers.']);

== matlab function Lib_Analytic/Solvers/Iterative NR Solver w JacobianCalc/NRwCond/Newton Raphson Solver/NR Update/Bounding/Throw Warning/MATLAB Function ==
  data: BlkNm_M parameter
function fcn(BlkNm_M)
%# Limit Newton Raphson outputs and produce a warning if it occurs
BName = BlkNm_M;
disp(['Warning in ' BName ': Solver limit has been hit, check for system convergence']);
